simulink model "h2p2_sim"  (R2022b)
settings: Solver=VariableStepAuto  StartTime=0.0  StopTime=Tf  RelTol=1e-3
undefined symbols (not defined in the file): h0, J, kd_pitch, kd_roll, kd_yaw, kp_pitch, kp_roll, kp_yaw, mu, n, q_inertial2body_0, r_inertial_0, v_inertial_0, w_b_0, w_b_nominal
libraries: matrix_library x1
settings Model: Creator=corey  LastModifiedBy=corey
settings DebuggingCC: UnconnectedInputMsg=warning  UnconnectedOutputMsg=warning  UnconnectedLineMsg=warning
settings ModelReferenceCC: EnableRefExpFcnMdlSchedulingChecks=on
settings RTWCC: DLArmComputeVersion=19.05

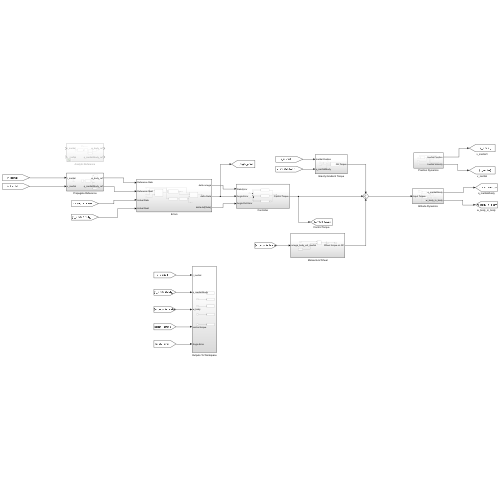
[thumbnail: Simulink's stored preview of the top-level diagram]
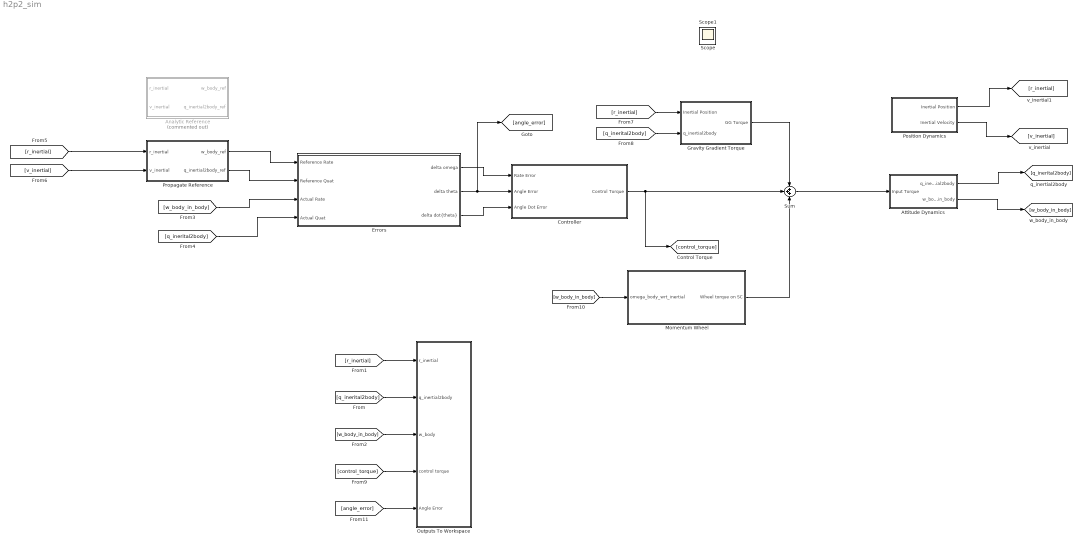
== system h2p2_sim ==
  Analytic Reference : Subsystem  Commented=on
  Attitude Dynamics : Subsystem
  Controller : Subsystem
  Errors : Subsystem
  Gravity Gradient Torque : Subsystem
  Momentum Wheel : Subsystem
  Outputs To Workspace : Subsystem
  Position Dynamics : Subsystem
  Propagate Reference : Subsystem
  Sum : Sum  Inputs=+++
  Scope : Scope
  Scope1 : Scope
  wires:
  Attitude Dynamics/2(w_body_in_body) -> [w_body_in_body]
  Gravity Gradient Torque/1(GG Torque) -> Sum/1
  Attitude Dynamics/1(q_inertial2body) -> [q_inerital2body]
  Position Dynamics/2(Inertial Velocity) -> [v_inertial]
  Position Dynamics/1(Inertial Position) -> [r_inertial]
  [q_inerital2body] -> Outputs To Workspace/2(q_inertial2body)
  [w_body_in_body] -> Outputs To Workspace/3(w_body)
  [r_inertial] -> Outputs To Workspace/1(r_inertial)
  Propagate Reference/1(w_body_ref) -> Errors/1(Reference Rate)
  Propagate Reference/2(q_inertial2body_ref) -> Errors/2(Reference Quat)
  [w_body_in_body] -> Errors/3(Actual Rate)
  [q_inerital2body] -> Errors/4(Actual Quat)
  [r_inertial] -> Propagate Reference/1(r_inertial)
  [v_inertial] -> Propagate Reference/2(v_inertial)
  [r_inertial] -> Gravity Gradient Torque/1(Inertial Position)
  [q_inerital2body] -> Gravity Gradient Torque/2(q_inertial2body)
  Errors/1(delta omega) -> Controller/1(Rate Error)
  Errors/2(delta theta) -> [angle_error], Controller/2(Angle Error)
  Errors/3("delta dot{theta}") -> Controller/3(Angle Dot Error)
  [control_torque] -> Outputs To Workspace/4(control torque)
  [w_body_in_body] -> Momentum Wheel/1(omega_body_wrt_inertial)
  Momentum Wheel/1(Wheel torque on SC) -> Sum/3
  Controller/1(Control Torque) -> Sum/2, [control_torque]
  [angle_error] -> Outputs To Workspace/5(Angle Error)
  Sum/1 -> Attitude Dynamics/1(Input Torque)

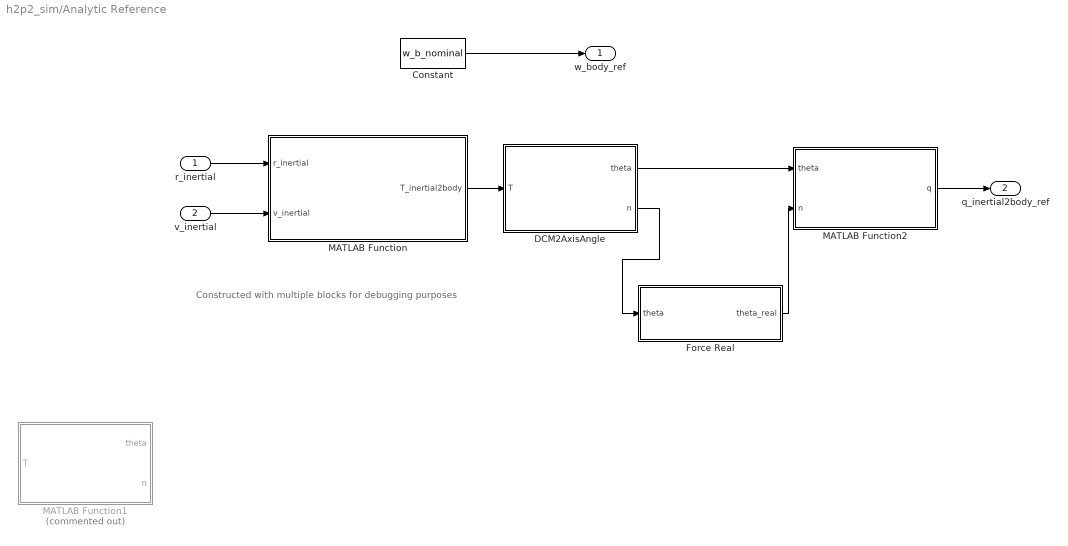
== system h2p2_sim/Analytic Reference ==
  note: Constructed with multiple blocks for debugging purposes
  r_inertial : Inport
  v_inertial : Inport  Port=2
  Constant : Constant  Value=w_b_nominal
  DCM2AxisAngle : Subsystem
  Force Real : MATLAB Function  TreatAsAtomicUnit=on
  MATLAB Function : MATLAB Function  TreatAsAtomicUnit=on
  MATLAB Function1 : MATLAB Function  Commented=on  TreatAsAtomicUnit=on
  MATLAB Function2 : MATLAB Function  TreatAsAtomicUnit=on
  w_body_ref : Outport
  q_inertial2body_ref : Outport  Port=2
  wires:
  v_inertial/1 -> MATLAB Function/2(v_inertial)
  r_inertial/1 -> MATLAB Function/1(r_inertial)
  Constant/1 -> w_body_ref/1
  MATLAB Function2/1(q) -> q_inertial2body_ref/1
  MATLAB Function/1(T_inertial2body) -> DCM2AxisAngle/1(T)
  DCM2AxisAngle/1(theta) -> MATLAB Function2/1(theta)
  DCM2AxisAngle/2(n) -> Force Real/1(theta)
  Force Real/1(theta_real) -> MATLAB Function2/2(n)

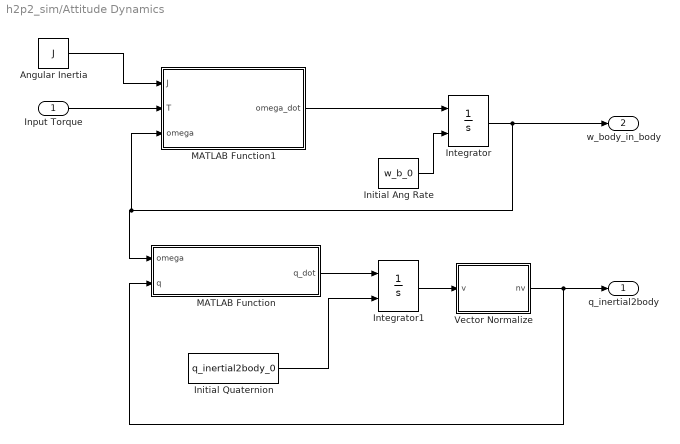
== system h2p2_sim/Attitude Dynamics ==
  Input Torque : Inport
  Angular Inertia : Constant  Value=J
  Initial Ang Rate : Constant  Value=w_b_0
  Initial Quaternion : Constant  Value=q_inertial2body_0
  Integrator : Integrator  InitialConditionSource=external
  Integrator1 : Integrator  InitialConditionSource=external
  MATLAB Function : MATLAB Function  TreatAsAtomicUnit=on
  MATLAB Function1 : MATLAB Function  TreatAsAtomicUnit=on
  Vector Normalize : MATLAB Function  TreatAsAtomicUnit=on
  q_inertial2body : Outport
  w_body_in_body : Outport  Port=2
  wires:
  Integrator/1 -> MATLAB Function1/3(omega), MATLAB Function/1(omega), w_body_in_body/1
  MATLAB Function1/1(omega_dot) -> Integrator/1
  Initial Ang Rate/1 -> Integrator/2
  MATLAB Function/1(q_dot) -> Integrator1/1
  Initial Quaternion/1 -> Integrator1/2
  Integrator1/1 -> Vector Normalize/1(v)
  Vector Normalize/1(nv) -> MATLAB Function/2(q), q_inertial2body/1
  Input Torque/1 -> MATLAB Function1/2(T)
  Angular Inertia/1 -> MATLAB Function1/1(J)

== system h2p2_sim/Controller ==
  Rate Error : Inport
  Angle Error : Inport  Port=2
  Angle Dot Error : Inport  Port=3
  Gain : Gain  Gain=0
  Mux : Mux  Inputs=3
  Pitch Loop : Subsystem
  Roll Loop : Subsystem
  Yaw Loop : Subsystem
  Control Torque : Outport
  wires:
  Angle Error/1 -> Pitch Loop/1(Angle Error), Roll Loop/1(Angle Error), Yaw Loop/1(Angle Error)
  Angle Dot Error/1 -> Pitch Loop/2(Angle Dot Error), Yaw Loop/2(Angle Dot Error), Roll Loop/2(Angle Dot Error)
  Roll Loop/1(Roll Angle Torque) -> Gain/1
  Mux/1 -> Control Torque/1
  Yaw Loop/1(Yaw Angle Torque) -> Mux/1
  Pitch Loop/1(Pitch Angle Torque) -> Mux/2
  Gain/1 -> Mux/3

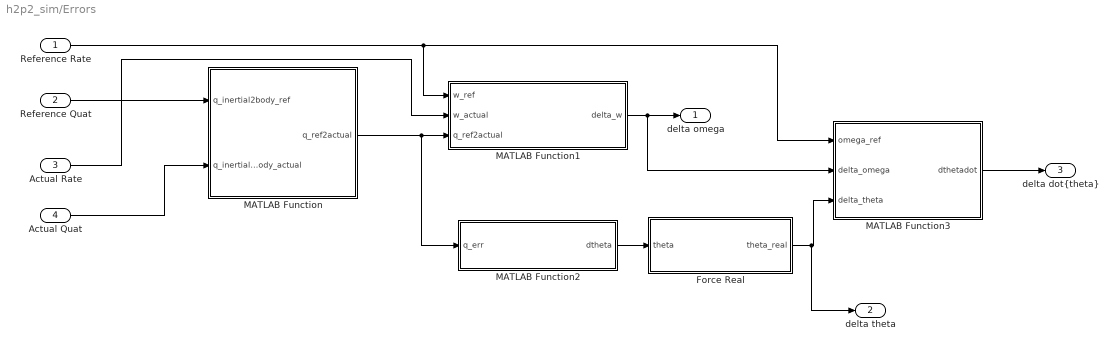
== system h2p2_sim/Errors ==
  Reference Rate : Inport
  Reference Quat : Inport  Port=2
  Actual Rate : Inport  Port=3
  Actual Quat : Inport  Port=4
  Force Real : MATLAB Function  TreatAsAtomicUnit=on
  MATLAB Function : MATLAB Function  TreatAsAtomicUnit=on
  MATLAB Function1 : MATLAB Function  TreatAsAtomicUnit=on
  MATLAB Function2 : MATLAB Function  TreatAsAtomicUnit=on
  MATLAB Function3 : MATLAB Function  TreatAsAtomicUnit=on
  delta omega : Outport
  delta theta : Outport  Port=2
  "delta dot{theta}" : Outport  Port=3
  wires:
  Reference Quat/1 -> MATLAB Function/1(q_inertial2body_ref)
  Actual Quat/1 -> MATLAB Function/2(q_inertial2body_actual)
  MATLAB Function/1(q_ref2actual) -> MATLAB Function2/1(q_err), MATLAB Function1/3(q_ref2actual)
  Reference Rate/1 -> MATLAB Function3/1(omega_ref), MATLAB Function1/1(w_ref)
  Actual Rate/1 -> MATLAB Function1/2(w_actual)
  MATLAB Function1/1(delta_w) -> MATLAB Function3/2(delta_omega), delta omega/1
  MATLAB Function3/1(dthetadot) -> "delta dot{theta}"/1
  MATLAB Function2/1(dtheta) -> Force Real/1(theta)
  Force Real/1(theta_real) -> delta theta/1, MATLAB Function3/3(delta_theta)

== system h2p2_sim/Gravity Gradient Torque ==
  Inertial Position : Inport
  q_inertial2body : Inport  Port=2
  GG Torque Computation : MATLAB Function  TreatAsAtomicUnit=on
  Gravity Constant : Constant  Value=mu
  Inerita Matrix : Constant  Value=J
  MATLAB Function : MATLAB Function  TreatAsAtomicUnit=on
  GG Torque : Outport
  wires:
  Inerita Matrix/1 -> GG Torque Computation/1(J)
  Inertial Position/1 -> MATLAB Function/2(r), GG Torque Computation/3(r_inertial)
  q_inertial2body/1 -> GG Torque Computation/4(q_inertial2body)
  GG Torque Computation/1(T) -> GG Torque/1
  Gravity Constant/1 -> MATLAB Function/1(mu)
  MATLAB Function/1(n) -> GG Torque Computation/2(n)

== system h2p2_sim/Momentum Wheel ==
  omega_body_wrt_inertial : Inport
  Constant : Constant  Value=[0 0 h0]'
  Cross Product : matrix_library/Cross Product
  Gain : Gain  Gain=-1
  Wheel torque on SC : Outport
  wires:
  omega_body_wrt_inertial/1 -> Cross Product/1
  Cross Product/1 -> Gain/1
  Gain/1 -> Wheel torque on SC/1
  Constant/1 -> Cross Product/2

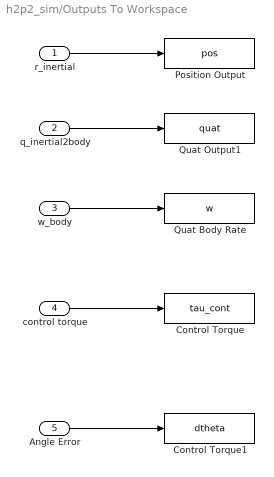
== system h2p2_sim/Outputs To Workspace ==
  r_inertial : Inport
  q_inertial2body : Inport  Port=2
  w_body : Inport  Port=3
  control torque : Inport  Port=4
  Angle Error : Inport  Port=5
  Control Torque : ToWorkspace  VariableName=tau_cont  SampleTime=-1
  Control Torque1 : ToWorkspace  VariableName=dtheta  SampleTime=-1
  Position Output : ToWorkspace  VariableName=pos  SampleTime=-1
  Quat Body Rate : ToWorkspace  VariableName=w  SampleTime=-1
  Quat Output1 : ToWorkspace  VariableName=quat  SampleTime=-1
  wires:
  r_inertial/1 -> Position Output/1
  w_body/1 -> Quat Body Rate/1
  q_inertial2body/1 -> Quat Output1/1
  control torque/1 -> Control Torque/1
  Angle Error/1 -> Control Torque1/1

== system h2p2_sim/Position Dynamics ==
  Gravity Constant : Constant  Value=mu
  Initial Position : Constant  Value=r_inertial_0
  Initial Velocity : Constant  Value=v_inertial_0
  Integrator : Integrator  InitialConditionSource=external  InitialCondition=[6871, 0, 0]'
  Integrator1 : Integrator  InitialConditionSource=external  InitialCondition=[0, 7.6166, 0]'
  Vector Norm : MATLAB Function  TreatAsAtomicUnit=on
  Inertial Position : Outport
  Inertial Velocity : Outport  Port=2
  wires:
  Integrator/1 -> Vector Norm/1(r), Inertial Position/1  "Position"
  Integrator1/1 -> Inertial Velocity/1, Integrator/1  "Velocity"
  Vector Norm/1(a) -> Integrator1/1  "Accel"
  Gravity Constant/1 -> Vector Norm/2(mu)
  Initial Velocity/1 -> Integrator1/2
  Initial Position/1 -> Integrator/2

== system h2p2_sim/Propagate Reference ==
  r_inertial : Inport
  v_inertial : Inport  Port=2
  Attitude Dynamics1 : Subsystem
  Constant : Constant  Value=[0 0 0]'
  To Workspace : ToWorkspace  VariableName=q_ref  SaveFormat=Timeseries  SampleTime=-1
  To Workspace1 : ToWorkspace  VariableName=w_ref  SaveFormat=Timeseries  SampleTime=-1
  w_body_ref : Outport
  q_inertial2body_ref : Outport  Port=2
  wires:
  Attitude Dynamics1/1(q_inertial2body) -> To Workspace/1, q_inertial2body_ref/1
  Attitude Dynamics1/2(w_body_in_body) -> To Workspace1/1, w_body_ref/1
  Constant/1 -> Attitude Dynamics1/1(Input Torque)

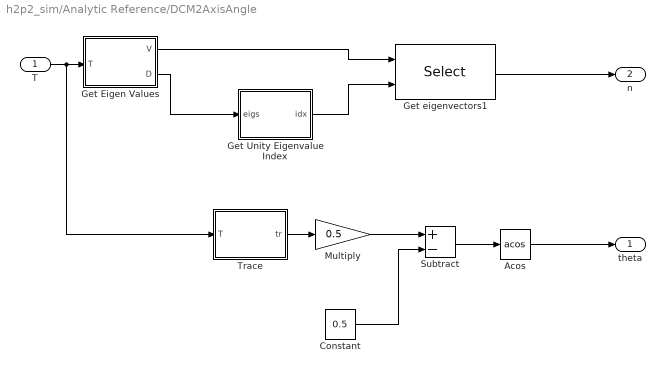
== system h2p2_sim/Analytic Reference/DCM2AxisAngle ==
  T : Inport
  Acos : Trigonometry  Operator=acos
  Constant : Constant  Value=0.5
  Get Eigen Values : MATLAB Function  TreatAsAtomicUnit=on
  Get Unity Eigenvalue Index : MATLAB Function  TreatAsAtomicUnit=on
  Get eigenvectors1 : Selector  NumberOfDimensions=2  InputPortWidth=3  IndexOptions=Index vector (dialog),Index vector (port)  Indices=[1 2 3],[1 2 3]  OutputSizes=1,1
  Multiply : Gain  Gain=0.5
  Subtract : Sum  Inputs=+-
  Trace : MATLAB Function  TreatAsAtomicUnit=on
  theta : Outport
  n : Outport  Port=2
  wires:
  T/1 -> Trace/1(T), Get Eigen Values/1(T)
  Get Eigen Values/1(V) -> Get eigenvectors1/1
  Get Eigen Values/2(D) -> Get Unity Eigenvalue Index/1(eigs)
  Get Unity Eigenvalue Index/1(idx) -> Get eigenvectors1/2
  Trace/1(tr) -> Multiply/1
  Multiply/1 -> Subtract/1
  Constant/1 -> Subtract/2
  Subtract/1 -> Acos/1
  Acos/1 -> theta/1
  Get eigenvectors1/1 -> n/1

== system h2p2_sim/Controller/Pitch Loop ==
  Angle Error : Inport
  Angle Dot Error : Inport  Port=2
  Add : Sum
  Cancellation Terms : Subsystem
  PD Controller : Subsystem
  Pitch Angle Torque : Outport
  wires:
  Add/1 -> Pitch Angle Torque/1
  Angle Error/1 -> Cancellation Terms/1(Angle Error), PD Controller/1(Angle Error)
  Angle Dot Error/1 -> Cancellation Terms/2(Angle Error Dot), PD Controller/2(Angle Error Dot)
  PD Controller/1(Out1) -> Add/2
  Cancellation Terms/1(Out1) -> Add/1

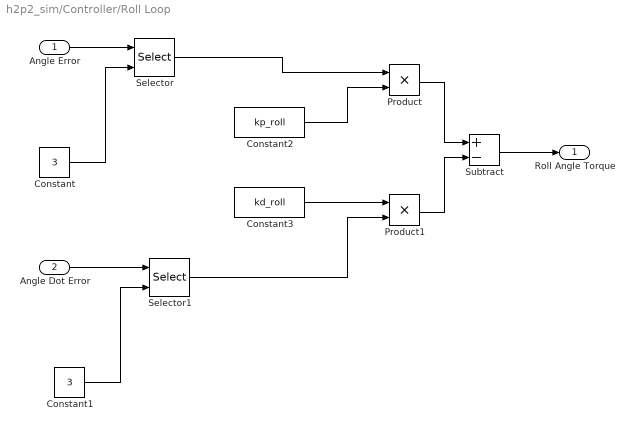
== system h2p2_sim/Controller/Roll Loop ==
  Angle Error : Inport
  Angle Dot Error : Inport  Port=2
  Constant : Constant  Value=3
  Constant1 : Constant  Value=3
  Constant2 : Constant  Value=kp_roll
  Constant3 : Constant  Value=kd_roll
  Product : Product
  Product1 : Product
  Selector : Selector  InputPortWidth=3  IndexOptions=Index vector (port)  Indices=[1 3]  OutputSizes=1
  Selector1 : Selector  InputPortWidth=3  IndexOptions=Index vector (port)  Indices=[1 3]  OutputSizes=1
  Subtract : Sum  Inputs=+-
  Roll Angle Torque : Outport
  wires:
  Angle Error/1 -> Selector/1
  Constant/1 -> Selector/2
  Constant1/1 -> Selector1/2
  Angle Dot Error/1 -> Selector1/1
  Selector/1 -> Product/1
  Constant2/1 -> Product/2
  Constant3/1 -> Product1/1
  Selector1/1 -> Product1/2
  Subtract/1 -> Roll Angle Torque/1
  Product/1 -> Subtract/1
  Product1/1 -> Subtract/2

== system h2p2_sim/Controller/Yaw Loop ==
  Angle Error : Inport
  Angle Dot Error : Inport  Port=2
  Add : Sum
  Cancellation Terms : Subsystem
  PD Controller : Subsystem
  Yaw Angle Torque : Outport
  wires:
  Add/1 -> Yaw Angle Torque/1
  Angle Error/1 -> Cancellation Terms/1(Angle Error), PD Controller/1(Angle Error)
  Angle Dot Error/1 -> Cancellation Terms/2(Angle Error Dot), PD Controller/2(Angle Error Dot)
  PD Controller/1(Out1) -> Add/2
  Cancellation Terms/1(Out1) -> Add/1

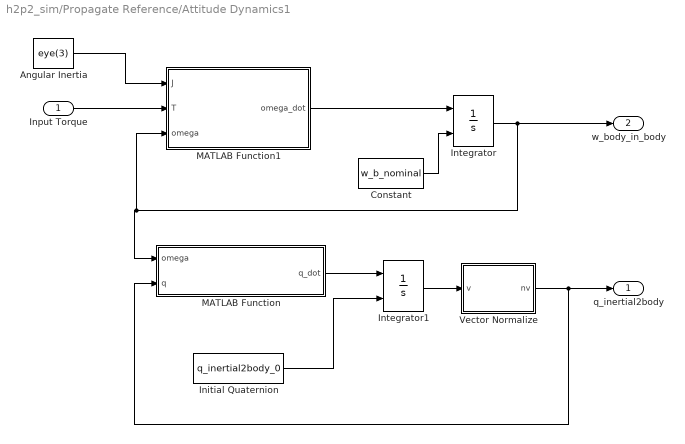
== system h2p2_sim/Propagate Reference/Attitude Dynamics1 ==
  Input Torque : Inport
  Angular Inertia : Constant  Value=eye(3)
  Constant : Constant  Value=w_b_nominal
  Initial Quaternion : Constant  Value=q_inertial2body_0
  Integrator : Integrator  InitialConditionSource=external
  Integrator1 : Integrator  InitialConditionSource=external
  MATLAB Function : MATLAB Function  TreatAsAtomicUnit=on
  MATLAB Function1 : MATLAB Function  TreatAsAtomicUnit=on
  Vector Normalize : MATLAB Function  TreatAsAtomicUnit=on
  q_inertial2body : Outport
  w_body_in_body : Outport  Port=2
  wires:
  Integrator/1 -> MATLAB Function1/3(omega), MATLAB Function/1(omega), w_body_in_body/1
  MATLAB Function1/1(omega_dot) -> Integrator/1
  Constant/1 -> Integrator/2
  MATLAB Function/1(q_dot) -> Integrator1/1
  Initial Quaternion/1 -> Integrator1/2
  Integrator1/1 -> Vector Normalize/1(v)
  Vector Normalize/1(nv) -> MATLAB Function/2(q), q_inertial2body/1
  Input Torque/1 -> MATLAB Function1/2(T)
  Angular Inertia/1 -> MATLAB Function1/1(J)

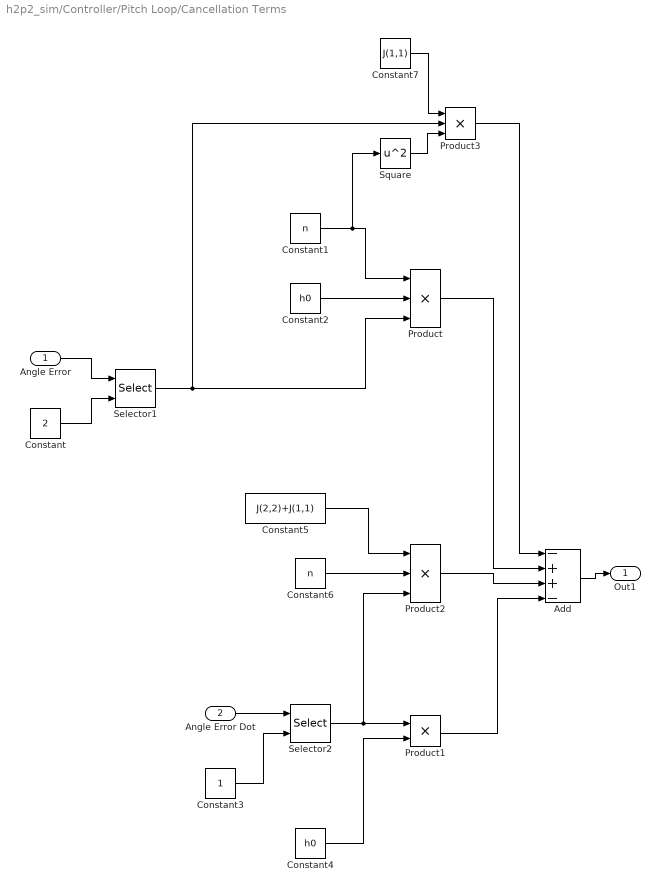
== system h2p2_sim/Controller/Pitch Loop/Cancellation Terms ==
  Angle Error : Inport
  Angle Error Dot : Inport  Port=2
  Add : Sum  Inputs=-++-
  Constant : Constant  Value=2
  Constant1 : Constant  Value=n
  Constant2 : Constant  Value=h0
  Constant3 : Constant
  Constant4 : Constant  Value=h0
  Constant5 : Constant  Value=J(2,2)+J(1,1)
  Constant6 : Constant  Value=n
  Constant7 : Constant  Value=J(1,1)
  Product : Product  Inputs=3
  Product1 : Product
  Product2 : Product  Inputs=3
  Product3 : Product  Inputs=3
  Selector1 : Selector  InputPortWidth=3  IndexOptions=Index vector (port)  Indices=[1 3]  OutputSizes=1
  Selector2 : Selector  InputPortWidth=3  IndexOptions=Index vector (port)  Indices=[1 3]  OutputSizes=1
  Square : Math  Operator=square
  Out1 : Outport
  wires:
  Angle Error/1 -> Selector1/1
  Constant/1 -> Selector1/2
  Selector1/1 -> Product3/2, Product/3
  Constant2/1 -> Product/2
  Constant1/1 -> Square/1, Product/1
  Angle Error Dot/1 -> Selector2/1
  Constant3/1 -> Selector2/2
  Selector2/1 -> Product2/3, Product1/1
  Constant4/1 -> Product1/2
  Constant6/1 -> Product2/2
  Constant5/1 -> Product2/1
  Add/1 -> Out1/1
  Product2/1 -> Add/3
  Product/1 -> Add/2
  Product1/1 -> Add/4
  Product3/1 -> Add/1
  Square/1 -> Product3/3
  Constant7/1 -> Product3/1

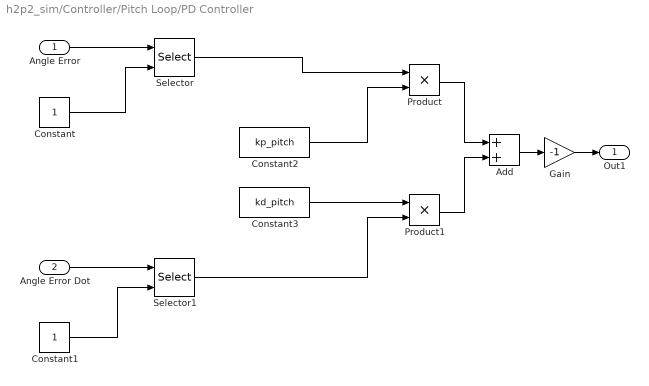
== system h2p2_sim/Controller/Pitch Loop/PD Controller ==
  Angle Error : Inport
  Angle Error Dot : Inport  Port=2
  Add : Sum
  Constant : Constant
  Constant1 : Constant
  Constant2 : Constant  Value=kp_pitch
  Constant3 : Constant  Value=kd_pitch
  Gain : Gain  Gain=-1
  Product : Product
  Product1 : Product
  Selector : Selector  InputPortWidth=3  IndexOptions=Index vector (port)  Indices=[1 3]  OutputSizes=1
  Selector1 : Selector  InputPortWidth=3  IndexOptions=Index vector (port)  Indices=[1 3]  OutputSizes=1
  Out1 : Outport
  wires:
  Constant2/1 -> Product/2
  Constant3/1 -> Product1/1
  Selector1/1 -> Product1/2
  Constant1/1 -> Selector1/2
  Angle Error Dot/1 -> Selector1/1
  Constant/1 -> Selector/2
  Product/1 -> Add/1
  Selector/1 -> Product/1
  Product1/1 -> Add/2
  Angle Error/1 -> Selector/1
  Add/1 -> Gain/1
  Gain/1 -> Out1/1

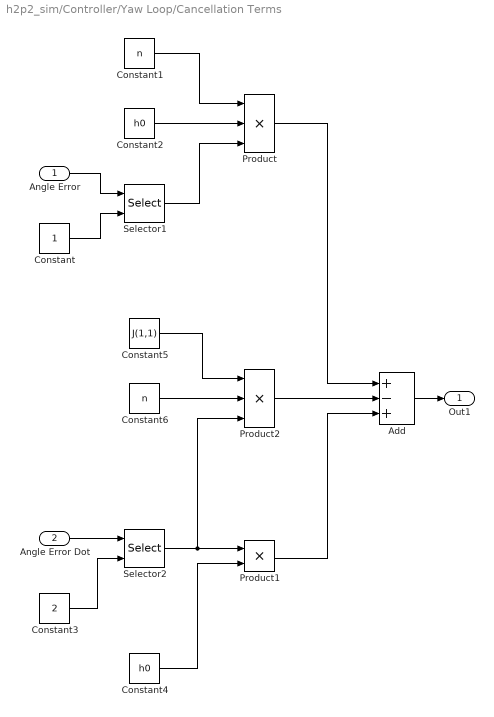
== system h2p2_sim/Controller/Yaw Loop/Cancellation Terms ==
  Angle Error : Inport
  Angle Error Dot : Inport  Port=2
  Add : Sum  Inputs=+-+
  Constant : Constant
  Constant1 : Constant  Value=n
  Constant2 : Constant  Value=h0
  Constant3 : Constant  Value=2
  Constant4 : Constant  Value=h0
  Constant5 : Constant  Value=J(1,1)
  Constant6 : Constant  Value=n
  Product : Product  Inputs=3
  Product1 : Product
  Product2 : Product  Inputs=3
  Selector1 : Selector  InputPortWidth=3  IndexOptions=Index vector (port)  Indices=[1 3]  OutputSizes=1
  Selector2 : Selector  InputPortWidth=3  IndexOptions=Index vector (port)  Indices=[1 3]  OutputSizes=1
  Out1 : Outport
  wires:
  Angle Error/1 -> Selector1/1
  Constant/1 -> Selector1/2
  Selector1/1 -> Product/3
  Constant2/1 -> Product/2
  Constant1/1 -> Product/1
  Angle Error Dot/1 -> Selector2/1
  Constant3/1 -> Selector2/2
  Selector2/1 -> Product2/3, Product1/1
  Constant4/1 -> Product1/2
  Constant6/1 -> Product2/2
  Constant5/1 -> Product2/1
  Add/1 -> Out1/1
  Product2/1 -> Add/2
  Product/1 -> Add/1
  Product1/1 -> Add/3

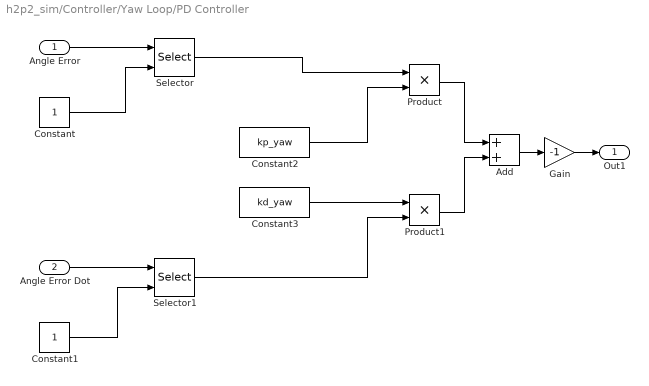
== system h2p2_sim/Controller/Yaw Loop/PD Controller ==
  Angle Error : Inport
  Angle Error Dot : Inport  Port=2
  Add : Sum
  Constant : Constant
  Constant1 : Constant
  Constant2 : Constant  Value=kp_yaw
  Constant3 : Constant  Value=kd_yaw
  Gain : Gain  Gain=-1
  Product : Product
  Product1 : Product
  Selector : Selector  InputPortWidth=3  IndexOptions=Index vector (port)  Indices=[1 3]  OutputSizes=1
  Selector1 : Selector  InputPortWidth=3  IndexOptions=Index vector (port)  Indices=[1 3]  OutputSizes=1
  Out1 : Outport
  wires:
  Constant2/1 -> Product/2
  Constant3/1 -> Product1/1
  Selector1/1 -> Product1/2
  Constant1/1 -> Selector1/2
  Angle Error Dot/1 -> Selector1/1
  Constant/1 -> Selector/2
  Product/1 -> Add/1
  Selector/1 -> Product/1
  Product1/1 -> Add/2
  Angle Error/1 -> Selector/1
  Add/1 -> Gain/1
  Gain/1 -> Out1/1

== matlab function h2p2_sim/Attitude Dynamics/MATLAB Function ==
  data: omega input; q_dot output; q input
function q_dot = QuaternionEvolution(omega, q)
intermed = [omega; 0];
q_dot = 0.5*QuatProduct(intermed,q);

== matlab function h2p2_sim/Propagate Reference/Attitude Dynamics1/MATLAB Function ==
  data: omega input; q_dot output; q input
function q_dot = QuaternionEvolution(omega, q)
intermed = [omega; 0];
q_dot = 0.5*QuatProduct(intermed,q);

== matlab function h2p2_sim/Propagate Reference/Attitude Dynamics1/MATLAB Function1 ==
  data: J input; omega_dot output; T input; omega input
function omega_dot = OmegaEvolution(J, T, omega)
omega_dot = J\(T - cross(omega, J*omega));

== matlab function h2p2_sim/Propagate Reference/Attitude Dynamics1/Vector Normalize ==
  data: v input; nv output
function nv = NormVec(v)

nv = v/norm(v);

== matlab function h2p2_sim/Analytic Reference/DCM2AxisAngle/Get Eigen Values ==
  data: T input; V output; D output
function [V, D] = eig_sim(T)

[V, D_mat] = eig(T);

% Get diagonals and only worry about real components
D = real(diag(D_mat));

== matlab function h2p2_sim/Analytic Reference/DCM2AxisAngle/Get Unity Eigenvalue Index ==
  data: eigs input; idx output
function idx = UnityEigIdx(eigs)

idxs = find(eigs == 1);

% if(length(idxs) > 1)
%     warning("More than one unity eigenvalue detected")
% end

if(length(idxs) < 1)
    idx = 1;
else
    idx = idxs(1);
end

== matlab function h2p2_sim/Analytic Reference/DCM2AxisAngle/Trace ==
  data: T input; tr output
function tr = Trace_sim(T)

tr = trace(T);

== matlab function h2p2_sim/Analytic Reference/Force Real ==
  data: theta input; theta_real output
function theta_real = ForceReal(theta)

theta_real = real(theta);

== matlab function h2p2_sim/Analytic Reference/MATLAB Function ==
  data: r_inertial input; T_inertial2body output; v_inertial input
function T_inertial2body = ConstructRefDCM(r_inertial, v_inertial)
% Construct nominal DCM

x_body_in_inertial = v_inertial/norm(v_inertial);
y_body_in_inertial = -r_inertial/norm(r_inertial);
z_body_in_inertial = cross(x_body_in_inertial,y_body_in_inertial);
T_inertial2body = [x_body_in_inertial';
    y_body_in_inertial';
    z_body_in_inertial'];

== matlab function h2p2_sim/Analytic Reference/MATLAB Function1 ==
  data: T input; theta output; n output
function [theta, n] = DCM2AxisAngle_sim(T)

[theta,n] = DCM2AxisAngle(T);

end

== matlab function h2p2_sim/Analytic Reference/MATLAB Function2 ==
  data: theta input; q output; n input
function q = AxisAngle2Quat_sim(theta,n)

q = AxisAngle2Quat(theta,n);

== matlab function h2p2_sim/Position Dynamics/Vector Norm ==
  data: r input; a output; mu input
function a = TwoBodyGrav(r,mu)

nr = norm(r);
a = -mu*r/(nr^3);

== matlab function h2p2_sim/Attitude Dynamics/MATLAB Function1 ==
  data: J input; omega_dot output; T input; omega input
function omega_dot = OmegaEvolution(J, T, omega)
omega_dot = J\(T - cross(omega, J*omega));

== matlab function h2p2_sim/Attitude Dynamics/Vector Normalize ==
  data: v input; nv output
function nv = NormVec(v)

nv = v/norm(v);

== matlab function h2p2_sim/Gravity Gradient Torque/GG Torque Computation ==
  data: J input; T output; n input; r_inertial input; q_inertial2body input
function T = GGTorque(J, n, r_inertial, q_inertial2body)

% Down in body frame
down_inertial = -r_inertial/norm(r_inertial);
down_body = QuatTransform(q_inertial2body,down_inertial);

% Gravity gradient torque
T = 3*n^2*cross(down_body,J*down_body);

== matlab function h2p2_sim/Gravity Gradient Torque/MATLAB Function ==
  data: mu input; n output; r input
function n = OrbitRate(mu,r)

n = sqrt(mu/norm(r)^3);

== matlab function h2p2_sim/Errors/MATLAB Function ==
  data: q_inertial2body_ref input; q_ref2actual output; q_inertial2body_actual input
function q_ref2actual = ErrorQuat(q_inertial2body_ref, q_inertial2body_actual)

q_ref2actual = QuatProduct(q_inertial2body_actual,QuatInv(q_inertial2body_ref));

% Force normalization
q_ref2actual = q_ref2actual/norm(q_ref2actual);

== matlab function h2p2_sim/Errors/MATLAB Function1 ==
  data: w_ref input; delta_w output; w_actual input; q_ref2actual input
function delta_w = ErrorRate(w_ref, w_actual, q_ref2actual)

delta_w = w_actual - QuatTransform(q_ref2actual,w_ref);

== matlab function h2p2_sim/Errors/MATLAB Function2 ==
  data: q_err input; dtheta output
function dtheta = ErrorQuat2ErrorAngle(q_err)

% Quaternion components
q_v = real(q_err(1:3));
q_s = real(q_err(4));

dtheta = [atan2(q_v(1),q_s);
    atan2(q_v(2),q_s);
    atan2(q_v(3),q_s)];

== matlab function h2p2_sim/Errors/MATLAB Function3 ==
  data: omega_ref input; dthetadot output; delta_omega input; delta_theta input
function dthetadot = ErrorThetaDot(omega_ref, delta_omega, delta_theta)

dthetadot = delta_omega - cross(omega_ref,delta_theta);

== matlab function h2p2_sim/Errors/Force Real ==
  data: theta input; theta_real output
function theta_real = ForceReal(theta)

theta_real = real(theta);
